simulink model "DYC_DLCtight_Fuzzy_and_NN_prediction"  (Simulink 8.9)
settings: Solver=VariableStepAuto  StartTime=0  StopTime=8  FixedStep=0.001  RelTol=1e-3  AbsTol=1e-6
libraries: neural x138, fuzblock x6, dspfdesign x6, Solver_SF x1, simulink x1
(part 4 of 4)

== system DYC_DLCtight_Fuzzy_and_NN_prediction/NN predictive optimized Fuzzy Control/6I6O Fitting Neural Network3/Layer 1/Delays 1 ==
  "p{1}" : Inport  PortDimensions=6
      mask Display: e = 0.06;c1 = [120 230 180]/255;c2 = ([120 230 180]+0)/(256+128);c3 = ([120 230 180]+128)/(256+128);patch([0 1 1 0],[0 0 1 1],c1);patch([0 1 1 1-e 1-e 0+e],[0 0 1 1-e 0+e 0+e],c2);patch([0 0 1 1-e 0+e 0+e],[0 1 1 1-e 1-e 0+e],c3);plot([0 1 1 0 0],[0 0 1 1 0]);
  mux : Mux  Inputs=1
      mask Display: e = 0.06;c1 = [120 150 230]/255;c2 = ([120 150 230]+0)/383;c3 = ([120 150 230]+128)/383;patch([0 1 1 0],[0 0 1 1],c1);patch([0 1 1 1-e 1-e 0+e],[0 0 1 1-e 0+e 0+e],c2);patch([0 0 1 1-e 0+e 0+e],[0 1 1 1-e 1-e 0+e],c3);plot([0 1 1 0 0],[0 0 1 1 0]);disp('Mux')
  "pd{1,1}" : Outport
      mask Display: e = 0.06;c1 = [120 230 180]/255;c2 = ([120 230 180]+0)/(256+128);c3 = ([120 230 180]+128)/(256+128);patch([0 1 1 0],[0 0 1 1],c1);patch([0 1 1 1-e 1-e 0+e],[0 0 1 1-e 0+e 0+e],c2);patch([0 0 1 1-e 0+e 0+e],[0 1 1 1-e 1-e 0+e],c3);plot([0 1 1 0 0],[0 0 1 1 0]);
  wires:
  "p{1}"/1 -> mux/1
  mux/1 -> "pd{1,1}"/1

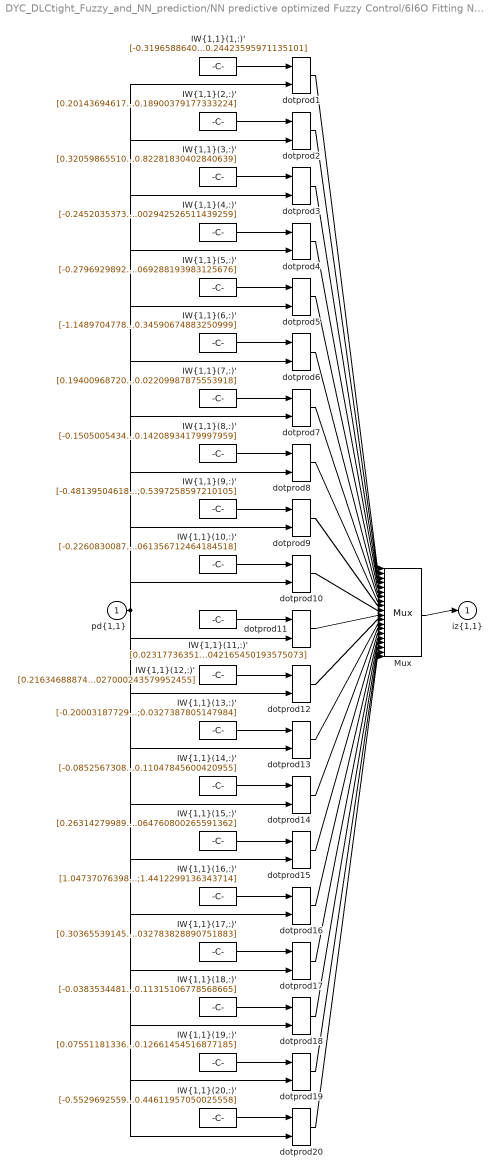
== system DYC_DLCtight_Fuzzy_and_NN_prediction/NN predictive optimized Fuzzy Control/6I6O Fitting Neural Network3/Layer 1/IW{1,1} ==
  "pd{1,1}" : Inport  PortDimensions=6
      mask Display: e = 0.06;c1 = [120 230 180]/255;c2 = ([120 230 180]+0)/(256+128);c3 = ([120 230 180]+128)/(256+128);patch([0 1 1 0],[0 0 1 1],c1);patch([0 1 1 1-e 1-e 0+e],[0 0 1 1-e 0+e 0+e],c2);patch([0 0 1 1-e 0+e 0+e],[0 1 1 1-e 1-e 0+e],c3);plot([0 1 1 0 0],[0 0 1 1 0]);
  "IW{1,1}(1,:)'" : Constant  Value=[-0.31965886406614341;0.052746311771913003;0.1045603514301662;-0.23936371643660831;-0.1544337035163153;0.24423595971135101]
      mask Display: e = 0.06;c1 = [120 150 230]/255;c2 = ([120 150 230]+0)/383;c3 = ([120 150 230]+128)/383;patch([0 1 1 0],[0 0 1 1],c1);patch([0 1 1 1-e 1-e 0+e],[0 0 1 1-e 0+e 0+e],c2);patch([0 0 1 1-e 0+e 0+e],[0 1 1 1-e 1-e 0+e],c3);plot([0 1 1 0 0],[0 0 1 1 0]);disp('Weights');
  "IW{1,1}(10,:)'" : Constant  Value=[-0.22608300874794299;-0.077216236992014756;0.01334322651626289;0.0039127938698336334;0.27607842671219557;0.061356712464184518]
      mask Display: e = 0.06;c1 = [120 150 230]/255;c2 = ([120 150 230]+0)/383;c3 = ([120 150 230]+128)/383;patch([0 1 1 0],[0 0 1 1],c1);patch([0 1 1 1-e 1-e 0+e],[0 0 1 1-e 0+e 0+e],c2);patch([0 0 1 1-e 0+e 0+e],[0 1 1 1-e 1-e 0+e],c3);plot([0 1 1 0 0],[0 0 1 1 0]);disp('Weights');
  "IW{1,1}(11,:)'" : Constant  Value=[0.02317736351236201;-0.021084097657146007;0.025368948160545392;0.023364108070201006;0.053995602057821737;0.0042165450193575073]
      mask Display: e = 0.06;c1 = [120 150 230]/255;c2 = ([120 150 230]+0)/383;c3 = ([120 150 230]+128)/383;patch([0 1 1 0],[0 0 1 1],c1);patch([0 1 1 1-e 1-e 0+e],[0 0 1 1-e 0+e 0+e],c2);patch([0 0 1 1-e 0+e 0+e],[0 1 1 1-e 1-e 0+e],c3);plot([0 1 1 0 0],[0 0 1 1 0]);disp('Weights');
  "IW{1,1}(12,:)'" : Constant  Value=[0.21634688874783833;-0.052760041247791836;-0.19424354064082378;-0.24541079567802876;-0.099328584948105647;0.0027000243579952455]
      mask Display: e = 0.06;c1 = [120 150 230]/255;c2 = ([120 150 230]+0)/383;c3 = ([120 150 230]+128)/383;patch([0 1 1 0],[0 0 1 1],c1);patch([0 1 1 1-e 1-e 0+e],[0 0 1 1-e 0+e 0+e],c2);patch([0 0 1 1-e 0+e 0+e],[0 1 1 1-e 1-e 0+e],c3);plot([0 1 1 0 0],[0 0 1 1 0]);disp('Weights');
  "IW{1,1}(13,:)'" : Constant  Value=[-0.20003187729155378;-0.078570755860069147;-0.018328280517202533;-0.03252656851336818;0.23166098986659409;0.0327387805147984]
      mask Display: e = 0.06;c1 = [120 150 230]/255;c2 = ([120 150 230]+0)/383;c3 = ([120 150 230]+128)/383;patch([0 1 1 0],[0 0 1 1],c1);patch([0 1 1 1-e 1-e 0+e],[0 0 1 1-e 0+e 0+e],c2);patch([0 0 1 1-e 0+e 0+e],[0 1 1 1-e 1-e 0+e],c3);plot([0 1 1 0 0],[0 0 1 1 0]);disp('Weights');
  "IW{1,1}(14,:)'" : Constant  Value=[-0.085256730842151837;0.063999042053410546;-0.049213457700109466;0.079379817070767369;0.036342672076749301;0.11047845600420955]
      mask Display: e = 0.06;c1 = [120 150 230]/255;c2 = ([120 150 230]+0)/383;c3 = ([120 150 230]+128)/383;patch([0 1 1 0],[0 0 1 1],c1);patch([0 1 1 1-e 1-e 0+e],[0 0 1 1-e 0+e 0+e],c2);patch([0 0 1 1-e 0+e 0+e],[0 1 1 1-e 1-e 0+e],c3);plot([0 1 1 0 0],[0 0 1 1 0]);disp('Weights');
  "IW{1,1}(15,:)'" : Constant  Value=[0.26314279989577588;-0.310761181601653;-0.055921090961742255;0.10477521658615613;-0.27291147706512481;0.064760800265591362]
      mask Display: e = 0.06;c1 = [120 150 230]/255;c2 = ([120 150 230]+0)/383;c3 = ([120 150 230]+128)/383;patch([0 1 1 0],[0 0 1 1],c1);patch([0 1 1 1-e 1-e 0+e],[0 0 1 1-e 0+e 0+e],c2);patch([0 0 1 1-e 0+e 0+e],[0 1 1 1-e 1-e 0+e],c3);plot([0 1 1 0 0],[0 0 1 1 0]);disp('Weights');
  "IW{1,1}(16,:)'" : Constant  Value=[1.0473707639882024;-0.26300980286969017;-0.78305714392097814;-0.30623459072851145;-0.21836628961644042;1.4412299136343714]
      mask Display: e = 0.06;c1 = [120 150 230]/255;c2 = ([120 150 230]+0)/383;c3 = ([120 150 230]+128)/383;patch([0 1 1 0],[0 0 1 1],c1);patch([0 1 1 1-e 1-e 0+e],[0 0 1 1-e 0+e 0+e],c2);patch([0 0 1 1-e 0+e 0+e],[0 1 1 1-e 1-e 0+e],c3);plot([0 1 1 0 0],[0 0 1 1 0]);disp('Weights');
  "IW{1,1}(17,:)'" : Constant  Value=[0.30365539145505049;-0.026051080977039967;0.028756839821146855;0.161217530619508;0.11380088084529806;0.032783828890751883]
      mask Display: e = 0.06;c1 = [120 150 230]/255;c2 = ([120 150 230]+0)/383;c3 = ([120 150 230]+128)/383;patch([0 1 1 0],[0 0 1 1],c1);patch([0 1 1 1-e 1-e 0+e],[0 0 1 1-e 0+e 0+e],c2);patch([0 0 1 1-e 0+e 0+e],[0 1 1 1-e 1-e 0+e],c3);plot([0 1 1 0 0],[0 0 1 1 0]);disp('Weights');
  "IW{1,1}(18,:)'" : Constant  Value=[-0.038353448179698581;0.094002225449665147;-0.056562441333226313;0.086135206486694788;-0.040573480772259744;0.11315106778568665]
      mask Display: e = 0.06;c1 = [120 150 230]/255;c2 = ([120 150 230]+0)/383;c3 = ([120 150 230]+128)/383;patch([0 1 1 0],[0 0 1 1],c1);patch([0 1 1 1-e 1-e 0+e],[0 0 1 1-e 0+e 0+e],c2);patch([0 0 1 1-e 0+e 0+e],[0 1 1 1-e 1-e 0+e],c3);plot([0 1 1 0 0],[0 0 1 1 0]);disp('Weights');
  "IW{1,1}(19,:)'" : Constant  Value=[0.075511813361896093;-0.08505263459563718;0.058671772993840167;-0.093589199419015043;-0.0087775159741800939;-0.12661454516877185]
      mask Display: e = 0.06;c1 = [120 150 230]/255;c2 = ([120 150 230]+0)/383;c3 = ([120 150 230]+128)/383;patch([0 1 1 0],[0 0 1 1],c1);patch([0 1 1 1-e 1-e 0+e],[0 0 1 1-e 0+e 0+e],c2);patch([0 0 1 1-e 0+e 0+e],[0 1 1 1-e 1-e 0+e],c3);plot([0 1 1 0 0],[0 0 1 1 0]);disp('Weights');
  "IW{1,1}(2,:)'" : Constant  Value=[0.20143694617419436;-0.094734967550365451;0.077367132223936597;-0.1145969189350102;-0.17348463672946079;0.18900379177333224]
      mask Display: e = 0.06;c1 = [120 150 230]/255;c2 = ([120 150 230]+0)/383;c3 = ([120 150 230]+128)/383;patch([0 1 1 0],[0 0 1 1],c1);patch([0 1 1 1-e 1-e 0+e],[0 0 1 1-e 0+e 0+e],c2);patch([0 0 1 1-e 0+e 0+e],[0 1 1 1-e 1-e 0+e],c3);plot([0 1 1 0 0],[0 0 1 1 0]);disp('Weights');
  "IW{1,1}(20,:)'" : Constant  Value=[-0.55296925594689361;-1.1384197800987041;-0.48523772949936483;-0.72981519585071863;1.0509708646676439;0.44611957050025558]
      mask Display: e = 0.06;c1 = [120 150 230]/255;c2 = ([120 150 230]+0)/383;c3 = ([120 150 230]+128)/383;patch([0 1 1 0],[0 0 1 1],c1);patch([0 1 1 1-e 1-e 0+e],[0 0 1 1-e 0+e 0+e],c2);patch([0 0 1 1-e 0+e 0+e],[0 1 1 1-e 1-e 0+e],c3);plot([0 1 1 0 0],[0 0 1 1 0]);disp('Weights');
  "IW{1,1}(3,:)'" : Constant  Value=[0.32059865510455021;0.66320666170297815;0.45495320964773245;-1.1455325908740221;-0.27891022836005946;0.82281830402840639]
      mask Display: e = 0.06;c1 = [120 150 230]/255;c2 = ([120 150 230]+0)/383;c3 = ([120 150 230]+128)/383;patch([0 1 1 0],[0 0 1 1],c1);patch([0 1 1 1-e 1-e 0+e],[0 0 1 1-e 0+e 0+e],c2);patch([0 0 1 1-e 0+e 0+e],[0 1 1 1-e 1-e 0+e],c3);plot([0 1 1 0 0],[0 0 1 1 0]);disp('Weights');
  "IW{1,1}(4,:)'" : Constant  Value=[-0.24520353739277789;0.059812661290350094;0.22148720092968763;0.27962202502336381;0.11300083400210405;-0.002942526511439259]
      mask Display: e = 0.06;c1 = [120 150 230]/255;c2 = ([120 150 230]+0)/383;c3 = ([120 150 230]+128)/383;patch([0 1 1 0],[0 0 1 1],c1);patch([0 1 1 1-e 1-e 0+e],[0 0 1 1-e 0+e 0+e],c2);patch([0 0 1 1-e 0+e 0+e],[0 1 1 1-e 1-e 0+e],c3);plot([0 1 1 0 0],[0 0 1 1 0]);disp('Weights');
  "IW{1,1}(5,:)'" : Constant  Value=[-0.27969298920639801;0.33133257110977843;0.059532167859124616;-0.11151364067814171;0.29000024717485812;-0.069288193983125676]
      mask Display: e = 0.06;c1 = [120 150 230]/255;c2 = ([120 150 230]+0)/383;c3 = ([120 150 230]+128)/383;patch([0 1 1 0],[0 0 1 1],c1);patch([0 1 1 1-e 1-e 0+e],[0 0 1 1-e 0+e 0+e],c2);patch([0 0 1 1-e 0+e 0+e],[0 1 1 1-e 1-e 0+e],c3);plot([0 1 1 0 0],[0 0 1 1 0]);disp('Weights');
  "IW{1,1}(6,:)'" : Constant  Value=[-1.1489704778060625;-0.80977023757061539;-0.32536333600132883;0.20829092373744587;-0.62711105584596794;0.34590674883250999]
      mask Display: e = 0.06;c1 = [120 150 230]/255;c2 = ([120 150 230]+0)/383;c3 = ([120 150 230]+128)/383;patch([0 1 1 0],[0 0 1 1],c1);patch([0 1 1 1-e 1-e 0+e],[0 0 1 1-e 0+e 0+e],c2);patch([0 0 1 1-e 0+e 0+e],[0 1 1 1-e 1-e 0+e],c3);plot([0 1 1 0 0],[0 0 1 1 0]);disp('Weights');
  "IW{1,1}(7,:)'" : Constant  Value=[0.19400968720607725;-0.013609761041849281;0.017135495394960034;0.10127863054647909;0.06409338341834836;0.02209987875553918]
      mask Display: e = 0.06;c1 = [120 150 230]/255;c2 = ([120 150 230]+0)/383;c3 = ([120 150 230]+128)/383;patch([0 1 1 0],[0 0 1 1],c1);patch([0 1 1 1-e 1-e 0+e],[0 0 1 1-e 0+e 0+e],c2);patch([0 0 1 1-e 0+e 0+e],[0 1 1 1-e 1-e 0+e],c3);plot([0 1 1 0 0],[0 0 1 1 0]);disp('Weights');
  "IW{1,1}(8,:)'" : Constant  Value=[-0.15050054345612637;0.070947284312131681;-0.058131521828810838;0.086374753782838237;0.12982485406663152;-0.14208934179997959]
      mask Display: e = 0.06;c1 = [120 150 230]/255;c2 = ([120 150 230]+0)/383;c3 = ([120 150 230]+128)/383;patch([0 1 1 0],[0 0 1 1],c1);patch([0 1 1 1-e 1-e 0+e],[0 0 1 1-e 0+e 0+e],c2);patch([0 0 1 1-e 0+e 0+e],[0 1 1 1-e 1-e 0+e],c3);plot([0 1 1 0 0],[0 0 1 1 0]);disp('Weights');
  "IW{1,1}(9,:)'" : Constant  Value=[-0.48139504618838891;-0.076335662299792106;0.81907367582075474;-1.4567147444509847;-1.5605843230028993;0.5397258597210105]
      mask Display: e = 0.06;c1 = [120 150 230]/255;c2 = ([120 150 230]+0)/383;c3 = ([120 150 230]+128)/383;patch([0 1 1 0],[0 0 1 1],c1);patch([0 1 1 1-e 1-e 0+e],[0 0 1 1-e 0+e 0+e],c2);patch([0 0 1 1-e 0+e 0+e],[0 1 1 1-e 1-e 0+e],c3);plot([0 1 1 0 0],[0 0 1 1 0]);disp('Weights');
  Mux : Mux  Inputs=20
      mask Display: e = 0.06;c1 = [120 150 230]/255;c2 = ([120 150 230]+0)/383;c3 = ([120 150 230]+128)/383;patch([0 1 1 0],[0 0 1 1],c1);patch([0 1 1 1-e 1-e 0+e],[0 0 1 1-e 0+e 0+e],c2);patch([0 0 1 1-e 0+e 0+e],[0 1 1 1-e 1-e 0+e],c3);plot([0 1 1 0 0],[0 0 1 1 0]);disp('Mux');
  dotprod{1..20} (20 alike) : neural/Weight Functions/dotprod
  "iz{1,1}" : Outport
      mask Display: e = 0.06;c1 = [120 230 180]/255;c2 = ([120 230 180]+0)/(256+128);c3 = ([120 230 180]+128)/(256+128);patch([0 1 1 0],[0 0 1 1],c1);patch([0 1 1 1-e 1-e 0+e],[0 0 1 1-e 0+e 0+e],c2);patch([0 0 1 1-e 0+e 0+e],[0 1 1 1-e 1-e 0+e],c3);plot([0 1 1 0 0],[0 0 1 1 0]);
  wires:
  "IW{1,1}(1,:)'"/1 -> dotprod1/1
  "pd{1,1}"/1 -> dotprod1/2, dotprod2/2, dotprod3/2, dotprod4/2, dotprod5/2, dotprod6/2, dotprod7/2, dotprod8/2, dotprod9/2, dotprod10/2, dotprod11/2, dotprod12/2, dotprod13/2, dotprod14/2, dotprod15/2, dotprod16/2, dotprod17/2, dotprod18/2, dotprod19/2, dotprod20/2
  dotprod1/1 -> Mux/1
  "IW{1,1}(2,:)'"/1 -> dotprod2/1
  dotprod2/1 -> Mux/2
  "IW{1,1}(3,:)'"/1 -> dotprod3/1
  dotprod3/1 -> Mux/3
  "IW{1,1}(4,:)'"/1 -> dotprod4/1
  dotprod4/1 -> Mux/4
  "IW{1,1}(5,:)'"/1 -> dotprod5/1
  dotprod5/1 -> Mux/5
  "IW{1,1}(6,:)'"/1 -> dotprod6/1
  dotprod6/1 -> Mux/6
  "IW{1,1}(7,:)'"/1 -> dotprod7/1
  dotprod7/1 -> Mux/7
  "IW{1,1}(8,:)'"/1 -> dotprod8/1
  dotprod8/1 -> Mux/8
  "IW{1,1}(9,:)'"/1 -> dotprod9/1
  dotprod9/1 -> Mux/9
  "IW{1,1}(10,:)'"/1 -> dotprod10/1
  dotprod10/1 -> Mux/10
  "IW{1,1}(11,:)'"/1 -> dotprod11/1
  dotprod11/1 -> Mux/11
  "IW{1,1}(12,:)'"/1 -> dotprod12/1
  dotprod12/1 -> Mux/12
  "IW{1,1}(13,:)'"/1 -> dotprod13/1
  dotprod13/1 -> Mux/13
  "IW{1,1}(14,:)'"/1 -> dotprod14/1
  dotprod14/1 -> Mux/14
  "IW{1,1}(15,:)'"/1 -> dotprod15/1
  dotprod15/1 -> Mux/15
  "IW{1,1}(16,:)'"/1 -> dotprod16/1
  dotprod16/1 -> Mux/16
  "IW{1,1}(17,:)'"/1 -> dotprod17/1
  dotprod17/1 -> Mux/17
  "IW{1,1}(18,:)'"/1 -> dotprod18/1
  dotprod18/1 -> Mux/18
  "IW{1,1}(19,:)'"/1 -> dotprod19/1
  dotprod19/1 -> Mux/19
  "IW{1,1}(20,:)'"/1 -> dotprod20/1
  dotprod20/1 -> Mux/20
  Mux/1 -> "iz{1,1}"/1

== system DYC_DLCtight_Fuzzy_and_NN_prediction/NN predictive optimized Fuzzy Control/6I6O Fitting Neural Network3/Layer 2/Delays 1 ==
  "p{2}" : Inport  PortDimensions=20
      mask Display: e = 0.06;c1 = [120 230 180]/255;c2 = ([120 230 180]+0)/(256+128);c3 = ([120 230 180]+128)/(256+128);patch([0 1 1 0],[0 0 1 1],c1);patch([0 1 1 1-e 1-e 0+e],[0 0 1 1-e 0+e 0+e],c2);patch([0 0 1 1-e 0+e 0+e],[0 1 1 1-e 1-e 0+e],c3);plot([0 1 1 0 0],[0 0 1 1 0]);
  mux : Mux  Inputs=1
      mask Display: e = 0.06;c1 = [120 150 230]/255;c2 = ([120 150 230]+0)/383;c3 = ([120 150 230]+128)/383;patch([0 1 1 0],[0 0 1 1],c1);patch([0 1 1 1-e 1-e 0+e],[0 0 1 1-e 0+e 0+e],c2);patch([0 0 1 1-e 0+e 0+e],[0 1 1 1-e 1-e 0+e],c3);plot([0 1 1 0 0],[0 0 1 1 0]);disp('Mux')
  "pd{2,1}" : Outport
      mask Display: e = 0.06;c1 = [120 230 180]/255;c2 = ([120 230 180]+0)/(256+128);c3 = ([120 230 180]+128)/(256+128);patch([0 1 1 0],[0 0 1 1],c1);patch([0 1 1 1-e 1-e 0+e],[0 0 1 1-e 0+e 0+e],c2);patch([0 0 1 1-e 0+e 0+e],[0 1 1 1-e 1-e 0+e],c3);plot([0 1 1 0 0],[0 0 1 1 0]);
  wires:
  "p{2}"/1 -> mux/1
  mux/1 -> "pd{2,1}"/1

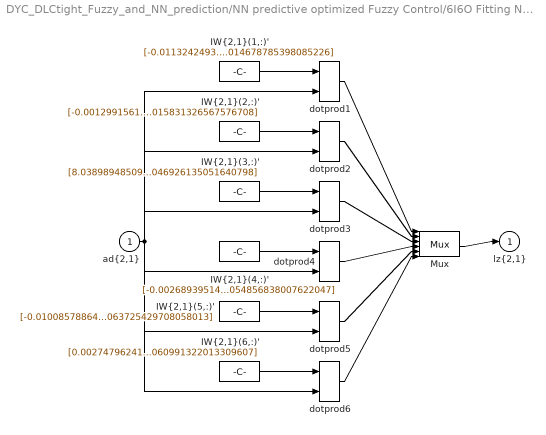
== system DYC_DLCtight_Fuzzy_and_NN_prediction/NN predictive optimized Fuzzy Control/6I6O Fitting Neural Network3/Layer 2/LW{2,1} ==
  "ad{2,1}" : Inport  PortDimensions=20
      mask Display: e = 0.06;c1 = [120 230 180]/255;c2 = ([120 230 180]+0)/(256+128);c3 = ([120 230 180]+128)/(256+128);patch([0 1 1 0],[0 0 1 1],c1);patch([0 1 1 1-e 1-e 0+e],[0 0 1 1-e 0+e 0+e],c2);patch([0 0 1 1-e 0+e 0+e],[0 1 1 1-e 1-e 0+e],c3);plot([0 1 1 0 0],[0 0 1 1 0]);
  "IW{2,1}(1,:)'" : Constant  Value=[-0.011324249341205796;0.15947337607203504;5.1892806272078789e-05;-0.67500730628936745;0.25623871631274581;0.00046016180601817804;2.3054630234784024;-0.23190751304055013;-4.2072784537522534e-06;0.65227154005334387;2.3684747287542631;0.88284542630217255;-1.847458086548653;-0.33682699498046431;-0.27980724741089924;-0.0001883471638795604;0.9190374325132985;-0.14258230659831431;0.34148575461810038;-0.014678785398085226]
      mask Display: e = 0.06;c1 = [120 150 230]/255;c2 = ([120 150 230]+0)/383;c3 = ([120 150 230]+128)/383;patch([0 1 1 0],[0 0 1 1],c1);patch([0 1 1 1-e 1-e 0+e],[0 0 1 1-e 0+e 0+e],c2);patch([0 0 1 1-e 0+e 0+e],[0 1 1 1-e 1-e 0+e],c3);plot([0 1 1 0 0],[0 0 1 1 0]);disp('weights');
  "IW{2,1}(2,:)'" : Constant  Value=[-0.0012991561131610911;0.017068966015925658;-0.00011655025594383416;-0.13915723901571611;1.4887273797114302;0.0001197267338686346;0.58733394023303209;-0.027114111085542278;1.2643393446893025e-05;-0.94448279559895065;-0.00089670749599506333;0.18203679883366036;-1.604127455974107;1.1381208342807483;-1.6863652507385187;9.4197978763726391e-05;0.22793777128445647;0.53287217723977753;-1.2604133008228269;-0.015831326567576708]
      mask Display: e = 0.06;c1 = [120 150 230]/255;c2 = ([120 150 230]+0)/383;c3 = ([120 150 230]+128)/383;patch([0 1 1 0],[0 0 1 1],c1);patch([0 1 1 1-e 1-e 0+e],[0 0 1 1-e 0+e 0+e],c2);patch([0 0 1 1-e 0+e 0+e],[0 1 1 1-e 1-e 0+e],c3);plot([0 1 1 0 0],[0 0 1 1 0]);disp('weights');
  "IW{2,1}(3,:)'" : Constant  Value=[8.0389894850968599e-05;1.6349507091194557;-0.0001933718487245591;1.676174730287439;0.74240016103842277;-9.6101013594233385e-05;-0.20007120803586767;-2.8890030628999814;1.8708399705022865e-05;-0.23684188967118616;1.4857209316141937;-2.1699941725969083;-0.33879144236411068;-1.8547231759627603;-0.84242549124308064;-0.0001842144734493714;-0.064110679368864568;-0.91677255287414416;2.0913667325622742;-0.0046926135051640798]
      mask Display: e = 0.06;c1 = [120 150 230]/255;c2 = ([120 150 230]+0)/383;c3 = ([120 150 230]+128)/383;patch([0 1 1 0],[0 0 1 1],c1);patch([0 1 1 1-e 1-e 0+e],[0 0 1 1-e 0+e 0+e],c2);patch([0 0 1 1-e 0+e 0+e],[0 1 1 1-e 1-e 0+e],c3);plot([0 1 1 0 0],[0 0 1 1 0]);disp('weights');
  "IW{2,1}(4,:)'" : Constant  Value=[-0.0026893951430255556;-1.1006026528475403;0.00010142665039412674;0.77643522273195187;-0.9391809597752101;0.00024437206218334525;0.97766541846244837;1.9544074454858362;-4.2489584896997381e-06;0.49925419179667074;0.84167283993697162;-1.0048011965707899;-1.4390617877235383;1.1255247837305578;1.0631076109057014;0.00016643771736190511;0.38760893893314385;0.54792879939247185;-1.2649637455063683;-0.0054856838007622047]
      mask Display: e = 0.06;c1 = [120 150 230]/255;c2 = ([120 150 230]+0)/383;c3 = ([120 150 230]+128)/383;patch([0 1 1 0],[0 0 1 1],c1);patch([0 1 1 1-e 1-e 0+e],[0 0 1 1-e 0+e 0+e],c2);patch([0 0 1 1-e 0+e 0+e],[0 1 1 1-e 1-e 0+e],c3);plot([0 1 1 0 0],[0 0 1 1 0]);disp('weights');
  "IW{2,1}(5,:)'" : Constant  Value=[-0.010085788641951485;-0.19336849206106022;4.7685683574392418e-05;-0.49877252764945945;0.60770998220135908;0.00044201186681115358;2.1146390479412878;0.38431338819150601;-3.8845474744871472e-06;1.5268247017384535;2.2932075347736536;0.65125896146079465;0.36465008255995041;-0.24863803200702217;-0.67905685595559373;-0.00012780739473478063;0.84342906512077531;-0.11033977941787927;0.25492154427720015;0.0063725429708058013]
      mask Display: e = 0.06;c1 = [120 150 230]/255;c2 = ([120 150 230]+0)/383;c3 = ([120 150 230]+128)/383;patch([0 1 1 0],[0 0 1 1],c1);patch([0 1 1 1-e 1-e 0+e],[0 0 1 1-e 0+e 0+e],c2);patch([0 0 1 1-e 0+e 0+e],[0 1 1 1-e 1-e 0+e],c3);plot([0 1 1 0 0],[0 0 1 1 0]);disp('weights');
  "IW{2,1}(6,:)'" : Constant  Value=[0.0027479624184045077;1.6434329903283726;-0.00012388304095788439;-0.10619810700297011;0.13724313250045642;0.0001422108289228424;0.37218895084668541;-2.914168107473559;2.3896472902831366e-06;1.6241903110698044;-0.59619830517671912;0.13527507008598272;-0.33973129401501212;2.0648210745334228;-0.15691687011152561;0.00024425094490209982;0.13555634949210979;1.0337530281977436;-2.3401348058648854;0.0060991322013309607]
      mask Display: e = 0.06;c1 = [120 150 230]/255;c2 = ([120 150 230]+0)/383;c3 = ([120 150 230]+128)/383;patch([0 1 1 0],[0 0 1 1],c1);patch([0 1 1 1-e 1-e 0+e],[0 0 1 1-e 0+e 0+e],c2);patch([0 0 1 1-e 0+e 0+e],[0 1 1 1-e 1-e 0+e],c3);plot([0 1 1 0 0],[0 0 1 1 0]);disp('weights');
  Mux : Mux  Inputs=6
      mask Display: e = 0.06;c1 = [120 150 230]/255;c2 = ([120 150 230]+0)/383;c3 = ([120 150 230]+128)/383;patch([0 1 1 0],[0 0 1 1],c1);patch([0 1 1 1-e 1-e 0+e],[0 0 1 1-e 0+e 0+e],c2);patch([0 0 1 1-e 0+e 0+e],[0 1 1 1-e 1-e 0+e],c3);plot([0 1 1 0 0],[0 0 1 1 0]);disp('Mux');
  dotprod{1..6} (6 alike) : neural/Weight Functions/dotprod
  "lz{2,1}" : Outport
      mask Display: e = 0.06;c1 = [120 230 180]/255;c2 = ([120 230 180]+0)/(256+128);c3 = ([120 230 180]+128)/(256+128);patch([0 1 1 0],[0 0 1 1],c1);patch([0 1 1 1-e 1-e 0+e],[0 0 1 1-e 0+e 0+e],c2);patch([0 0 1 1-e 0+e 0+e],[0 1 1 1-e 1-e 0+e],c3);plot([0 1 1 0 0],[0 0 1 1 0]);
  wires:
  "IW{2,1}(1,:)'"/1 -> dotprod1/1
  "ad{2,1}"/1 -> dotprod1/2, dotprod2/2, dotprod3/2, dotprod4/2, dotprod5/2, dotprod6/2
  dotprod1/1 -> Mux/1
  "IW{2,1}(2,:)'"/1 -> dotprod2/1
  dotprod2/1 -> Mux/2
  "IW{2,1}(3,:)'"/1 -> dotprod3/1
  dotprod3/1 -> Mux/3
  "IW{2,1}(4,:)'"/1 -> dotprod4/1
  dotprod4/1 -> Mux/4
  "IW{2,1}(5,:)'"/1 -> dotprod5/1
  dotprod5/1 -> Mux/5
  "IW{2,1}(6,:)'"/1 -> dotprod6/1
  dotprod6/1 -> Mux/6
  Mux/1 -> "lz{2,1}"/1

== matlab function Station PID/ PID speed control method ==
  data: BrakeTorque output double; Vd input double; Vx input double; station input double; Vd_o input double

function BrakeTorque  = Speed_Control(Vd, Vx, station, Vd_o)  %(Fz_fl, Fz_rl, Fz_fr, Fz_rr,M_dyc,delta)

        if station>-5 && station < 55   %减小Vx以缩小横摆半径，有利于提高避障能力。
            BrakeTorque =20*(Vd-Vx);
        else
            BrakeTorque = 10*(Vd_o-Vx);
        end

end

== matlab function DYC Control/DYC  control method ==
  data: T1 output double; T2 output double; T3 output double; T4 output double; delta input double; beta input double; Fz_fl input double; Fz_fr input double; Fz_rl input double; Fz_rr input double

function [T1,T2,T3,T4] = DYC_Control(delta,beta,Fz_fl, Fz_fr, Fz_rl, Fz_rr)  %(Fz_fl, Fz_rl, Fz_fr, Fz_rr,M_dyc,delta)

       R = 0.347;
       tw_f = 1.845;
       tw_r = 1.845;
       a = 1.050;
       
       Fz = Fz_fl + Fz_fr + Fz_rl + Fz_rr;
%         T1p = (Fz_fl / Fz) * M_dyc * R / (-1 * tw_f / 2 * cos(delta) + a * sin(delta));
%         T2p = (Fz_fr / Fz) * M_dyc * R / (tw_f /2 * cos(delta) + a * sin(delta));
%         T3p = (Fz_rl / Fz) * M_dyc * R / (2*tw_r);
%         T4p = (Fz_rr / Fz) * M_dyc * R / (2*tw_r);
       if abs(beta) < 4 % 当质心侧偏角比较小的时候，考虑提供直接横摆力矩，提高转向能力
           M_dyc = 10*abs(delta);
            if delta < 0
                T1 =  (Fz_fl / Fz) * M_dyc * R/ (-1 * tw_f / 2 * cos(delta*pi/180) + a * sin(delta*pi/180));
                T2 = -(Fz_fr / Fz) * M_dyc * R / (tw_f /2 * cos(delta*pi/180) + a * sin(delta*pi/180));
                T3 = (Fz_rl / Fz) * M_dyc * R / (2*tw_r);
                T4 = -(Fz_rr / Fz) * M_dyc * R / (2*tw_r);
            else
                T1 =  -(Fz_fl / Fz) * M_dyc * R / (-1 * tw_f / 2 * cos(delta*pi/180) + a * sin(delta*pi/180));
                T2 = (Fz_fr / Fz) * M_dyc * R / (tw_f /2 * cos(delta*pi/180) + a * sin(delta*pi/180));
                T3 = -(Fz_rl / Fz) * M_dyc * R / (2*tw_r);
                T4 = (Fz_rr / Fz) * M_dyc * R / (2*tw_r);
            end
       else  %当质心侧偏角比较大的时候，考虑调整车速姿态，缩小汽车的质心侧偏角，保持侧向稳定。
           M_dyc = 20*abs(delta);
            if beta < 0
                T1 =  (Fz_fl / Fz) * M_dyc * R/ (-1 * tw_f / 2 * cos(delta*pi/180) + a * sin(delta*pi/180));
                T2 = -(Fz_fr / Fz) * M_dyc * R / (tw_f /2 * cos(delta*pi/180) + a * sin(delta*pi/180));
                T3 = (Fz_rl / Fz) * M_dyc * R / (2*tw_r);
                T4 = -(Fz_rr / Fz) * M_dyc * R / (2*tw_r);
            else
                T1 =  -(Fz_fl / Fz) * M_dyc * R / (-1 * tw_f / 2 * cos(delta*pi/180) + a * sin(delta*pi/180));
                T2 = (Fz_fr / Fz) * M_dyc * R / (tw_f /2 * cos(delta*pi/180) + a * sin(delta*pi/180));
                T3 = -(Fz_rl / Fz) * M_dyc * R / (2*tw_r);
                T4 = (Fz_rr / Fz) * M_dyc * R / (2*tw_r);
            end 
            
       end
       
%        if abs(delta) >3  %减小Vx以缩小横摆半径，有利于提高避障能力。
%             BrakeForce = 5*abs(delta);
%             T1 = T1 - Tspeed;
%             T2 = T2 - Tspeed;
%             T3 = T3 - Tspeed;
%             T4 = T4 - Tspeed;
%       end
end
%         f rintf('所需的四个力矩分别为：%f  %f  %f  %f \n', T1, T2, T3, T4);

== matlab function Fuzzy_Vd ==
  data: Fuzzy_Vd output double; Actual_Mu input double

function Fuzzy_Vd  = Fuzzy_Vd(Actual_Mu)  %(Fz_fl, Fz_rl, Fz_fr, Fz_rr,M_dyc,delta)

 sigma = 0.06; %width
 Mu = [0.2   0.4   0.6   0.8   1]; %centers
    x =  [15   28    35    48   55]; 
% x = (0.0:0.01:1.2)'; 
% y1 = exp(-(x - Mu(1)).^2/(2*sigma^2));
% y2 = exp(-(x - Mu(2)).^2/(2*sigma^2));
% y3 = exp(-(x - Mu(3)).^2/(2*sigma^2));
% y4 = exp(-(x - Mu(4)).^2/(2*sigma^2));
% y5 = exp(-(x - Mu(5)).^2/(2*sigma^2));
% 
% figure (21);
% plot(x, [y1 y2 y3 y4 y5]); 

y1 = exp(-(Actual_Mu - Mu(1)).^2/(2*sigma^2));
y2 = exp(-(Actual_Mu - Mu(2)).^2/(2*sigma^2));
y3 = exp(-(Actual_Mu - Mu(3)).^2/(2*sigma^2));
y4 = exp(-(Actual_Mu - Mu(4)).^2/(2*sigma^2));
y5 = exp(-(Actual_Mu - Mu(5)).^2/(2*sigma^2));

y = [y1 y2 y3 y4 y5];  %fprintf('\n the coefficients are:\n\n [%f, %f, %f, %f, %f]\n\n\n',y);

y =y / sum(y); %归一化
 
Fuzzy_Vd = x * y';  

end

== matlab function NN predictive optimized Fuzzy Control/Select Vd ==
  data: Vd input double; Ve output double; Vx input double; station input double; Vd_o input double; Vd_r output double
function [Ve, Vd_r]  = select(Vd, Vx, station, Vd_o)  %(Fz_fl, Fz_rl, Fz_fr, Fz_rr,M_dyc,delta)

        if station>-5 && station < 55   %减小Vx以缩小横摆半径，有利于提高避障能力。
            Ve =Vd-Vx;
            Vd_r = Vd;
        else
            Ve = Vd_o-Vx;
            Vd_r = Vd_o;
        end

end

== matlab function  Fuzzy Control/Select Vd ==
  data: Vd input double; Ve output double; Vx input double; station input double; Vd_o input double
function Ve  = select(Vd, Vx, station, Vd_o)  %(Fz_fl, Fz_rl, Fz_fr, Fz_rr,M_dyc,delta)

        if station>-5 && station < 55   %减小Vx以缩小横摆半径，有利于提高避障能力。
            Ve =Vd-Vx;
        else
            Ve = Vd_o-Vx;
        end

end

== matlab function Increment PID /Select Vd ==
  data: Vd input double; Ve output double; Vx input double; station input double; Vd_o input double
function Ve  = select(Vd, Vx, station, Vd_o)  %(Fz_fl, Fz_rl, Fz_fr, Fz_rr,M_dyc,delta)

        if station>-5 && station < 55   %减小Vx以缩小横摆半径，有利于提高避障能力。
            Ve =Vd-Vx;
        else
            Ve = Vd_o-Vx;
        end

end

== matlab function NN predictive optimized Fuzzy Control/MATLAB Function ==
  data: O_PID input double; Ve input double; Force output double; O_MPC input double
function Force = SignalSelection(O_PID, Ve, O_MPC)
  
  if abs(Ve) > 0.1
      Force = O_MPC;
  else
      Force = O_PID;
  end

end
